simulink model "dc_motor_ideal_voltage_with_controller"  (R2019b)
settings: Solver=VariableStepAuto  StartTime=0.0  StopTime=400  FixedStep=1  RelTol=1e-6
settings Model: NumberOfSteps=5  SnapshotInterval=1  Creator=srikesh  LastModifiedBy=srikesh
settings SolverCC: ZeroCrossAlgorithm=Adaptive
settings DebuggingCC: IgnoredZcDiagnostic=none

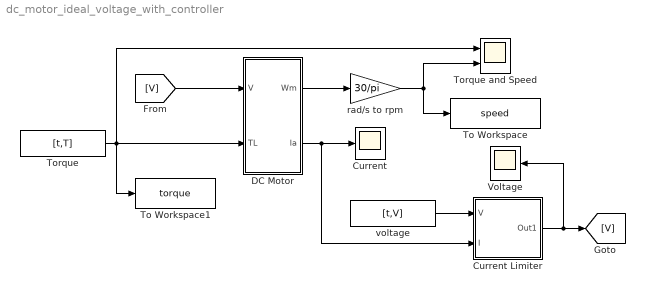
== system dc_motor_ideal_voltage_with_controller ==
  Current : Scope
  Current Limiter : Subsystem
  "DC Motor " : Subsystem  mask{Ra=.1472, Ke=1.27, Kt=.9852, J=.01, b=.005}
      mask prompts: Ra "Ra(Ohm)"; Ke "Ke(V-s)"; Kt "Kt(N-m/A)"; J "J(kg-m^2)"; b "b(N-m-s)"
  To Workspace : ToWorkspace  VariableName=speed  SaveFormat=Timeseries  SampleTime=-1
  To Workspace1 : ToWorkspace  VariableName=torque  SaveFormat=Timeseries  SampleTime=-1
  "Torque " : FromWorkspace  VariableName=[t,T]  SampleTime=0
  Torque and Speed : Scope  NumInputPorts=2
  Voltage : Scope
  "rad/s to rpm " : Gain  Gain=30/pi
  voltage : FromWorkspace  VariableName=[t,V]  SampleTime=0
  wires:
  "DC Motor "/1("Wm ") -> "rad/s to rpm "/1
  "rad/s to rpm "/1 -> To Workspace/1, Torque and Speed/2
  "DC Motor "/2(Ia) -> Current Limiter/2(I), Current/1
  "Torque "/1 -> Torque and Speed/1, "DC Motor "/2("TL "), To Workspace1/1
  [V] -> "DC Motor "/1("V ")
  Current Limiter/1(Out1) -> Voltage/1, [V]
  voltage/1 -> Current Limiter/1(V)

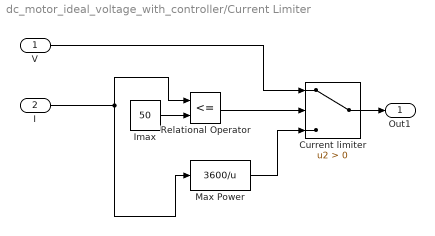
== system dc_motor_ideal_voltage_with_controller/Current Limiter ==
  V : Inport
  I : Inport  Port=2
  "Current limiter " : Switch  Criteria=u2 > Threshold
  Imax : Constant  Value=50
  Max Power : Fcn  Expr=3600/u
  Relational Operator : RelationalOperator  Operator=<=  OutDataTypeStr=boolean  RndMeth=Simplest
  Out1 : Outport
  wires:
  V/1 -> "Current limiter "/1
  "Current limiter "/1 -> Out1/1
  Max Power/1 -> "Current limiter "/3
  I/1 -> Relational Operator/1, Max Power/1
  Imax/1 -> Relational Operator/2
  Relational Operator/1 -> "Current limiter "/2

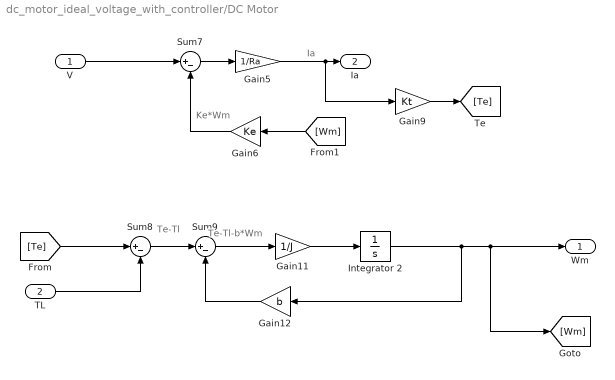
== system dc_motor_ideal_voltage_with_controller/DC Motor  ==
  note: Te-Tl-b*Wm
  note: Te-Tl
  note: Ia
  note: Ke*Wm
  "V " : Inport
  "TL " : Inport  Port=2
  Gain11 : Gain  Gain=1/J
  Gain12 : Gain  Gain=b
  Gain5 : Gain  Gain=1/Ra
  Gain6 : Gain  Gain=Ke
  Gain9 : Gain  Gain=Kt
  Integrator 2 : Integrator
  Sum7 : Sum  Inputs=|+-
  Sum8 : Sum  Inputs=|+-
  Sum9 : Sum  Inputs=|+-
  "Wm " : Outport
  Ia : Outport  Port=2
  wires:
  "V "/1 -> Sum7/1
  Gain6/1 -> Sum7/2
  Gain12/1 -> Sum9/2
  [Te] -> Sum8/1
  [Wm] -> Gain6/1
  Sum8/1 -> Sum9/1
  Gain9/1 -> [Te]
  "TL "/1 -> Sum8/2
  Gain11/1 -> Integrator 2/1
  Sum9/1 -> Gain11/1
  Integrator 2/1 -> Gain12/1, "Wm "/1, [Wm]
  Sum7/1 -> Gain5/1
  Gain5/1 -> Gain9/1, Ia/1
